simulink model "es4_sim"  (Simulink 7.9)
settings: Solver=ode45  StartTime=0.0  StopTime=10.0  RelTol=1e-3
values from neighbouring files (symbols this model uses):
  A = [3 -2;-7 3]    [es4.m]
  B = [1;3]    [es4.m]
  C = [1 1]    [es4.m]
  K = place(A,B,autoval)    [es4.m]
  L = place(A',C',10*autoval)'    [es4.m]
  x0 = [1 1]    [es4.m]
  xeq = -inv(A)*B*ueq    [es4.m]
undefined symbols (not defined in the file or in its folder): ueq
settings Model: Creator=claudio  LastModifiedBy=patrizio
settings OptimizationCC: InlineInvariantSignals=on  InitFltsAndDblsToZero=on
settings DebuggingCC: SaveWithParameterizedLinksMsg=none  SignalResolutionControl=TryResolveAllWithWarning  MultiTaskDSMMsg=warning  MultiTaskCondExecSysMsg=none  FcnCallInpInsideContextMsg=Use local settings  StrictBusMsg=None
settings RTWCC: IncludeERTFirstTime=on
settings GRTTargetCC: TargetFcnLib=ansi_tfl_tmw.mat  CombineOutputUpdateFcns=off  GRTInterface=on

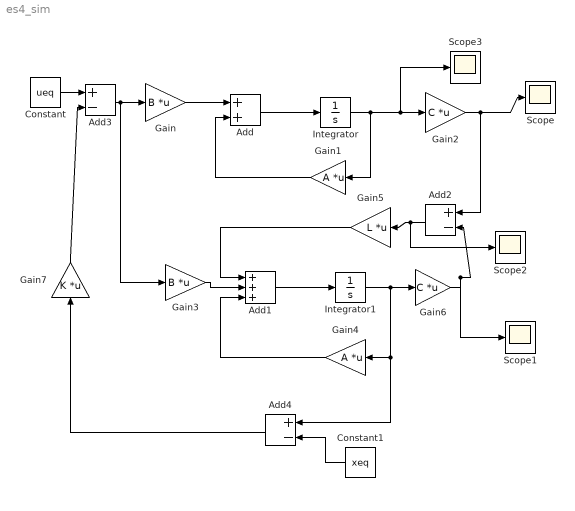
== system es4_sim ==
  Add : Sum
  Add1 : Sum  Inputs=+++
  Add2 : Sum  Inputs=+-
  Add3 : Sum  Inputs=+-
  Add4 : Sum  Inputs=+-
  Constant : Constant  Value=ueq
  Constant1 : Constant  Value=xeq
  Gain : Gain  Gain=B  Multiplication=Matrix(K*u)
  Gain1 : Gain  Gain=A  Multiplication=Matrix(K*u)
  Gain2 : Gain  Gain=C  Multiplication=Matrix(K*u)
  Gain3 : Gain  Gain=B  Multiplication=Matrix(K*u)
  Gain4 : Gain  Gain=A  Multiplication=Matrix(K*u)
  Gain5 : Gain  Gain=L  Multiplication=Matrix(K*u)
  Gain6 : Gain  Gain=C  Multiplication=Matrix(K*u)
  Gain7 : Gain  Gain=K  Multiplication=Matrix(K*u)
  Integrator : Integrator  InitialCondition=x0
  Integrator1 : Integrator
  Scope{,1..3} (4 alike) : Scope
      Scope2 settings: SaveName=ScopeData2
      Scope3 settings: SaveName=ScopeData3
  wires:
  Add/1 -> Integrator/1
  Gain/1 -> Add/1
  Integrator/1 -> Gain1/1, Gain2/1, Scope3/1
  Gain1/1 -> Add/2
  Add1/1 -> Integrator1/1
  Integrator1/1 -> Gain6/1, Gain4/1, Add4/1
  Gain2/1 -> Add2/1, Scope/1
  Add2/1 -> Gain5/1, Scope2/1
  Gain5/1 -> Add1/1
  Gain3/1 -> Add1/2
  Gain4/1 -> Add1/3
  Gain6/1 -> Add2/2, Scope1/1
  Add3/1 -> Gain/1, Gain3/1
  Constant/1 -> Add3/1
  Gain7/1 -> Add3/2
  Constant1/1 -> Add4/2
  Add4/1 -> Gain7/1
